simulink model "Mdl_8"  (R2017b)
settings: Solver=ode4  StartTime=0.0  StopTime=10000  FixedStep=0.01  RelTol=1e-3
undefined symbols (not defined in the file): Cg, Cs, k, kc, kg, kr, simSwitch, u0, v0, x0
settings Model: Creator=lasse  LastModifiedBy=lasse
settings DataIOCC: SaveFinalState=on  SaveFormat=StructureWithTime  SaveState=on  SignalLogging=off  DSMLogging=off

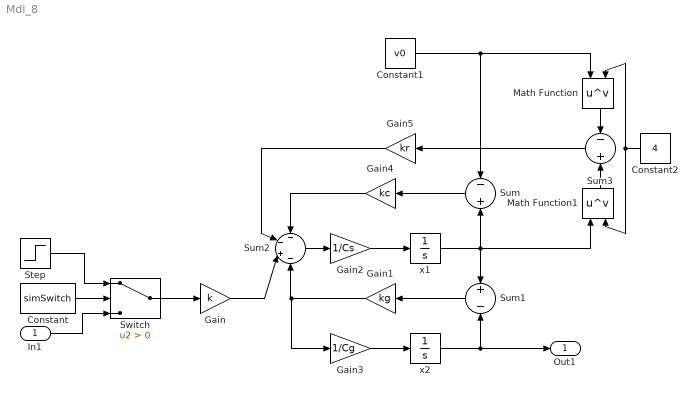
== system Mdl_8 ==
  In1 : Inport
  Constant : Constant  Value=simSwitch
  Constant1 : Constant  Value=v0
  Constant2 : Constant  Value=4
  Gain : Gain  Gain=k
  Gain1 : Gain  Gain=kg
  Gain2 : Gain  Gain=1/Cs
  Gain3 : Gain  Gain=1/Cg
  Gain4 : Gain  Gain=kc
  Gain5 : Gain  Gain=kr
  Math Function : Math  Operator=pow  SaturateOnIntegerOverflow=on
  Math Function1 : Math  Operator=pow  SaturateOnIntegerOverflow=on
  Step : Step  Time=0  Before=u0  After=u0  SampleTime=0
  Sum : Sum  Inputs=-+
  Sum1 : Sum  Inputs=+-
  Sum2 : Sum  Inputs=--+-
  Sum3 : Sum  Inputs=-+
  Switch : Switch  Criteria=u2 > Threshold
  x1 : Integrator  Priority=1  InitialCondition=x0(1)
  x2 : Integrator  Priority=2  InitialCondition=x0(2)
  Out1 : Outport
  wires:
  Constant/1 -> Switch/2
  In1/1 -> Switch/3
  Step/1 -> Switch/1
  Switch/1 -> Gain/1
  x2/1 -> Out1/1, Sum1/2
  x1/1 -> Math Function1/1, Sum1/1, Sum/2
  Sum1/1 -> Gain1/1
  Gain2/1 -> x1/1
  Gain3/1 -> x2/1
  Sum2/1 -> Gain2/1
  Gain1/1 -> Gain3/1, Sum2/4
  Gain/1 -> Sum2/3
  Sum/1 -> Gain4/1
  Constant1/1 -> Math Function/1, Sum/1
  Gain4/1 -> Sum2/1
  Math Function1/1 -> Sum3/2
  Math Function/1 -> Sum3/1
  Constant2/1 -> Math Function/2, Math Function1/2
  Sum3/1 -> Gain5/1
  Gain5/1 -> Sum2/2
